simulink model "model_spis"  (R2016b)
settings: Solver=FixedStepDiscrete  StartTime=0.0  StopTime=inf  FixedStep=sampleTime  RelTol=1e-3
PostLoadFcn:
  | parameters_spis;
  | 
  | % set requested state
  | set_param('model_spis/Requested state','Value',num2str(0));
InitFcn:
  | parameters_spis;
  | 
  | % set requested state
  | set_param('model_spis/Requested state','Value',num2str(0));
StartFcn:
  | parameters_spis;
  | 
  | % set requested state
  | set_param('model_spis/Requested state','Value',num2str(0));
undefined symbols (not defined in the file): FM1, FM2, Lb, Lf, Lu, sampleTime
libraries: simulink x29, LibraryFM x14, VariousBlocksLibrary x7, simulink_extras x1
(part 3 of 3)

== matlab function model_spis/Experiment & Haptics/Subsystem3/visuomotor rotation1 ==
  data: xBound input; pos_ref output; yBound input; vel input; pos_ref_prev input; sampleTime parameter; vel_ref output
function [pos_ref, vel_ref] = rotation(xBound, yBound, vel, pos_ref_prev,sampleTime)

persistent velDir;

if isempty(velDir)
    velDir = [1;0]; % initial velocity
end

pos_ref_tmp = pos_ref_prev + velDir*vel*sampleTime;

% check for x boundary
if (pos_ref_tmp(1) > xBound)
    velDir = [0;1];
elseif (pos_ref_tmp(1) < -xBound)
    velDir = [0;-1];
elseif (pos_ref_tmp(2) > yBound)
    velDir = [-1;0];
elseif (pos_ref_tmp(2) < -yBound)
    velDir = [1;0];
end

% forward Euler integration
pos_ref = pos_ref_prev + velDir*vel*sampleTime;
vel_ref = velDir*vel;

end

== matlab function model_spis/Robot1/DataFromEtherCAT/Calculate Arrange Joint and Op Space/forward kinematics1/Je ==
  data: q input; Je output size=[2 2]; Lf parameter; Lu parameter; Lb parameter
function Je = Je( q, Lf, Lu, Lb)
%#codegen

% Calculate the Jacobian for this particular device configuration.
% Note that the function func_eq_Je needs to be in the libraries/kinematis_functions folder

% jacobians
Je = func_eq_Je(q(1),q(2),Lf,Lu,Lb);

== matlab function model_spis/Robot1/DataFromEtherCAT/Calculate Arrange Joint and Op Space/forward kinematics1/Jedot ==
  data: q input; qdot input; Jedot output size=[2 2]; Lf parameter; Lu parameter; Lb parameter
function Jedot = Jedot( q, qdot, Lf, Lu, Lb)
%#codegen

% Calculate the time derivative of the Jacobian for this particular device configuration.
% Note that the function func_eq_Je needs to be in the libraries/kinematis_functions folder


% jacobians
Jedot = func_eq_Jedot(q(1),q(2),qdot(1),qdot(2),Lf,Lu,Lb);

== matlab function model_spis/Robot1/DataFromEtherCAT/Calculate Arrange Joint and Op Space/forward kinematics1/calculate xddot ==
  data: qddot input; qdot input size=[2 1]; J input; xddot output size=[2 1]; Jdot input
function xddot = calc_xddot(qddot, qdot, J, Jdot)
%#codegen

xddot = J*qddot + Jdot*qdot;

== matlab function model_spis/Robot2/Controller_PD/PD + nonlin (op space)/nonlinear compensation ==
  data: J input; Jdot input; qdot input; tau output; RobotStruct parameter
function tau = n(J,Jdot,qdot,RobotStruct)
% mass matrix
phat = RobotStruct.DynModParams;

% select parameters
me = phat(3);
Fs1 = phat(4);
Fv1 = phat(5);
Fs2 = phat(6);
Fv2 = phat(7);

% % jacobians
% J = func_eq_Je(q(1),q(2),Lf,Lu,Lb);
% Jdot = func_eq_Jedot(q(1),q(2),qdot(1),qdot(2),Lf,Lu,Lb);

% calculate joint space mass matrix;
p = [me;Fs1;Fv1;Fs2;Fv2];

% psi 
Psi = [(J'*Jdot)*qdot [ssign(qdot(1)) qdot(1); 0 0] [0 0; ssign(qdot(2)) qdot(2)]];

% torque
tau = Psi*p;

function x = ssign(u,b)
%% x = ssign(u,b)
% soft sign
if nargin < 2
    b = 4;
end

x = 2./(1+exp(-b*u))-1;

== matlab function model_spis/Experiment & Haptics/visuomotor rotation ==
  data: x_home input; x input; y output; theta input; doRotation input
function y = fcn(x_home,x,theta,doRotation)

x = x - x_home;

if (doRotation)
    R = [cos(theta) -sin(theta); 
         sin(theta) cos(theta)];
    y = R*x;
else
    y = x;
end

y = y + x_home;

== matlab function model_spis/Robot1/DataFromEtherCAT/Calculate Arrange Joint and Op Space/forward kinematics/forward kinematics ==
  data: q input; x output size=[2 1]; Lf parameter; Lu parameter; Lb parameter
function x = FK(q, Lf, Lu, Lb)
%#codegen

% Calculate the endpoint position (forward kinematics)
% Note that the function func_eq_FK needs to be in the libraries/kinematis_functions folder


x = func_eq_FK(q(1),q(2),Lf,Lu,Lb);

== matlab function model_spis/Robot1/DataFromEtherCAT/Calculate Arrange Joint and Op Space/forward kinematics1/forward kinematics ==
  data: q input; x output size=[2 1]; Lf parameter; Lu parameter; Lb parameter
function x = FK(q, Lf, Lu, Lb)
%#codegen

% Calculate the endpoint position (forward kinematics)
% Note that the function func_eq_FK needs to be in the libraries/kinematis_functions folder


x = func_eq_FK(q(1),q(2),Lf,Lu,Lb);

== matlab function model_spis/Robot1/DataToEtherCAT/FTSensorError/MATLAB Function ==
  data: ForcesTorques input; e output; MaxForcesTorques input
function e = fcn(ForcesTorques, MaxForcesTorques)

% throw error when any of the forces/torques go over a max allowable value
if any(abs(ForcesTorques) > MaxForcesTorques) 
    e = 1;
else
    e = 0;
end

== matlab function model_spis/Robot1/Controller_PD/PD + nonlin (op space)/invJ1 ==
  data: x input; J input; y output
function y = invJ(x,J)

y = J.'*x;

== matlab function model_spis/Robot2/DataFromEtherCAT/Calculate Arrange Joint and Op Space/Condition number ==
  data: J input; C output
function C = conditioning(J)
%#codegen

C = norm(J)*norm(pinv(J));

== matlab function model_spis/Robot2/DataFromEtherCAT/Calculate Arrange Joint and Op Space/IK all joints ==
  data: x input; q_all output; Lf parameter; Lu parameter; Lb parameter
function q_all = IK_all(x,Lf,Lu,Lb)
%#codegen

q_all = func_eqs_IK_all(x(1),x(2),Lf,Lu,Lb);

if any(isnan(q_all)) || any(isinf(q_all))
    q_all = zeros(5,1);
end

== matlab function model_spis/Robot2/DataFromEtherCAT/Calculate Arrange Joint and Op Space/forward kinematics/Je ==
  data: q input; Je output size=[2 2]; Lf parameter; Lu parameter; Lb parameter
function Je = Je( q, Lf, Lu, Lb)
%#codegen

% Calculate the Jacobian for this particular device configuration.
% Note that the function func_eq_Je needs to be in the libraries/kinematis_functions folder

% jacobians
Je = func_eq_Je(q(1),q(2),Lf,Lu,Lb);

== matlab function model_spis/Experiment & Haptics/visuomotor rotation1 ==
  data: x_home input; x input; y output; theta input; doRotation input
function y = fcn(x_home,x,theta,doRotation)

x = x - x_home;

if (doRotation)
    R = [cos(theta) -sin(theta); 
         sin(theta) cos(theta)];
    y = R*x;
else
    y = x;
end

y = y + x_home;

== matlab function model_spis/Robot2/DataFromEtherCAT/Calculate Arrange Joint and Op Space/forward kinematics/Jedot ==
  data: q input; qdot input; Jedot output size=[2 2]; Lf parameter; Lu parameter; Lb parameter
function Jedot = Jedot( q, qdot, Lf, Lu, Lb)
%#codegen

% Calculate the time derivative of the Jacobian for this particular device configuration.
% Note that the function func_eq_Je needs to be in the libraries/kinematis_functions folder


% jacobians
Jedot = func_eq_Jedot(q(1),q(2),qdot(1),qdot(2),Lf,Lu,Lb);

== matlab function model_spis/Robot1/DataFromEtherCAT/Calculate Arrange Joint and Op Space/forward kinematics/Je ==
  data: q input; Je output size=[2 2]; Lf parameter; Lu parameter; Lb parameter
function Je = Je( q, Lf, Lu, Lb)
%#codegen

% Calculate the Jacobian for this particular device configuration.
% Note that the function func_eq_Je needs to be in the libraries/kinematis_functions folder

% jacobians
Je = func_eq_Je(q(1),q(2),Lf,Lu,Lb);

== matlab function model_spis/Robot1/DataFromEtherCAT/Calculate Arrange Joint and Op Space/forward kinematics/Jedot ==
  data: q input; qdot input; Jedot output size=[2 2]; Lf parameter; Lu parameter; Lb parameter
function Jedot = Jedot( q, qdot, Lf, Lu, Lb)
%#codegen

% Calculate the time derivative of the Jacobian for this particular device configuration.
% Note that the function func_eq_Je needs to be in the libraries/kinematis_functions folder


% jacobians
Jedot = func_eq_Jedot(q(1),q(2),qdot(1),qdot(2),Lf,Lu,Lb);

== matlab function model_spis/Robot1/DataFromEtherCAT/FTSensor_K6D27/CorrectOffset ==
  data: u_in input; u_out output; reset input; corrected output
function [u_out,corrected] = CorrectOffset(u_in,reset)
%#codegen

persistent data_ offset_ counter_ corrected_;
N = 1000;

% initialize
if isempty(data_)
    data_ = zeros(size(u_in,1), N);
    offset_ = zeros(size(u_in));
    counter_ = 1;
    corrected_ = 0;
end

if (counter_ <= N)
    data_(:,counter_) = u_in;
end

counter_ = counter_ + 1;
if reset
    counter_ = 1;
end

% calculate mean
if counter_ == N
    corrected_ = 1;
    offset_ = mean(data_,2);
end

corrected = corrected_;
u_out = u_in - offset_;

== matlab function model_spis/Robot2/DataFromEtherCAT/Calculate Arrange Joint and Op Space/forward kinematics/calculate xddot ==
  data: qddot input; qdot input size=[2 1]; J input; xddot output size=[2 1]; Jdot input
function xddot = calc_xddot(qddot, qdot, J, Jdot)
%#codegen

xddot = J*qddot + Jdot*qdot;

== matlab function model_spis/Robot1/DataFromEtherCAT/Calculate Arrange Joint and Op Space/IK all joints ==
  data: x input; q_all output; Lf parameter; Lu parameter; Lb parameter
function q_all = IK_all(x,Lf,Lu,Lb)
%#codegen

q_all = func_eqs_IK_all(x(1),x(2),Lf,Lu,Lb);

if any(isnan(q_all)) || any(isinf(q_all))
    q_all = zeros(5,1);
end

== matlab function model_spis/Robot1/DataFromEtherCAT/Calculate Arrange Joint and Op Space/forward kinematics/calculate xddot ==
  data: qddot input; qdot input size=[2 1]; J input; xddot output size=[2 1]; Jdot input
function xddot = calc_xddot(qddot, qdot, J, Jdot)
%#codegen

xddot = J*qddot + Jdot*qdot;

== matlab function model_spis/Robot2/DataFromEtherCAT/Calculate Arrange Joint and Op Space/forward kinematics/forward kinematics ==
  data: q input; x output size=[2 1]; Lf parameter; Lu parameter; Lb parameter
function x = FK(q, Lf, Lu, Lb)
%#codegen

% Calculate the endpoint position (forward kinematics)
% Note that the function func_eq_FK needs to be in the libraries/kinematis_functions folder


x = func_eq_FK(q(1),q(2),Lf,Lu,Lb);

== matlab function model_spis/Robot1/Controller_PD/PD + nonlin (op space)/nonlinear compensation ==
  data: J input; Jdot input; qdot input; tau output; RobotStruct parameter
function tau = n(J,Jdot,qdot,RobotStruct)
% mass matrix
phat = RobotStruct.DynModParams;

% select parameters
me = phat(3);
Fs1 = phat(4);
Fv1 = phat(5);
Fs2 = phat(6);
Fv2 = phat(7);

% % jacobians
% J = func_eq_Je(q(1),q(2),Lf,Lu,Lb);
% Jdot = func_eq_Jedot(q(1),q(2),qdot(1),qdot(2),Lf,Lu,Lb);

% calculate joint space mass matrix;
p = [me;Fs1;Fv1;Fs2;Fv2];

% psi 
Psi = [(J'*Jdot)*qdot [ssign(qdot(1)) qdot(1); 0 0] [0 0; ssign(qdot(2)) qdot(2)]];

% torque
tau = Psi*p;

function x = ssign(u,b)
%% x = ssign(u,b)
% soft sign
if nargin < 2
    b = 8;
end

x = 2./(1+exp(-b*u))-1;

== matlab function model_spis/Robot2/DataFromEtherCAT/Calculate Arrange Joint and Op Space/forward kinematics1/Je ==
  data: q input; Je output size=[2 2]; Lf parameter; Lu parameter; Lb parameter
function Je = Je( q, Lf, Lu, Lb)
%#codegen

% Calculate the Jacobian for this particular device configuration.
% Note that the function func_eq_Je needs to be in the libraries/kinematis_functions folder

% jacobians
Je = func_eq_Je(q(1),q(2),Lf,Lu,Lb);

== matlab function model_spis/Robot2/DataFromEtherCAT/Calculate Arrange Joint and Op Space/forward kinematics1/Jedot ==
  data: q input; qdot input; Jedot output size=[2 2]; Lf parameter; Lu parameter; Lb parameter
function Jedot = Jedot( q, qdot, Lf, Lu, Lb)
%#codegen

% Calculate the time derivative of the Jacobian for this particular device configuration.
% Note that the function func_eq_Je needs to be in the libraries/kinematis_functions folder


% jacobians
Jedot = func_eq_Jedot(q(1),q(2),qdot(1),qdot(2),Lf,Lu,Lb);

== matlab function model_spis/Robot2/DataFromEtherCAT/Calculate Arrange Joint and Op Space/forward kinematics1/calculate xddot ==
  data: qddot input; qdot input size=[2 1]; J input; xddot output size=[2 1]; Jdot input
function xddot = calc_xddot(qddot, qdot, J, Jdot)
%#codegen

xddot = J*qddot + Jdot*qdot;

== matlab function model_spis/Robot2/DataFromEtherCAT/Calculate Arrange Joint and Op Space/forward kinematics1/forward kinematics ==
  data: q input; x output size=[2 1]; Lf parameter; Lu parameter; Lb parameter
function x = FK(q, Lf, Lu, Lb)
%#codegen

% Calculate the endpoint position (forward kinematics)
% Note that the function func_eq_FK needs to be in the libraries/kinematis_functions folder


x = func_eq_FK(q(1),q(2),Lf,Lu,Lb);

== matlab function model_spis/Robot2/DataFromEtherCAT/FTSensor_K6D27/CorrectOffset ==
  data: u_in input; u_out output; reset input; corrected output
function [u_out,corrected] = CorrectOffset(u_in,reset)
%#codegen

persistent data_ offset_ counter_ corrected_;
N = 1000;

% initialize
if isempty(data_)
    data_ = zeros(size(u_in,1), N);
    offset_ = zeros(size(u_in));
    counter_ = 1;
    corrected_ = 0;
end

if (counter_ <= N)
    data_(:,counter_) = u_in;
end

counter_ = counter_ + 1;
if reset
    counter_ = 1;
end

% calculate mean
if counter_ == N
    corrected_ = 1;
    offset_ = mean(data_,2);
end

corrected = corrected_;
u_out = u_in - offset_;

== matlab function model_spis/Experiment & Haptics/isAtTarget ==
  data: cursorPos input; atTarget output; targetPos input
function atTarget = isAtTarget(cursorPos, targetPos)

if (norm(cursorPos-targetPos) < 0.003)
    atTarget = 1;
else
    atTarget = 0;
end

== matlab function model_spis/Robot2/DataFromEtherCAT/FTSensor_K6D27/SensorToOperationalSpace ==
  data: q_all input; Fs input; FTOpSpace output; transmatside input
function FTOpSpace = ForceSensorToOperationalSpace(q_all,Fs,transmatside)
%#codegen
q1 = q_all(1);
q2 = q_all(2);
q4 = q_all(4);
q5 = q_all(5);

% based on which arm the force sensor is connected
switch transmatside
    case 1
        alpha = pi-q2;   
        beta = q1+alpha-pi/2;
        R0 = rotmat(beta);
        R = blkdiag(R0,R0); % transform forces and moments
    case 2
        alpha = -(pi - q4);
        beta = q5+alpha-pi/2;
        R0 = rotmat(beta);
        R = blkdiag(R0,R0); % transform forces and moments
    otherwise
        R = eye(length(Fs));
end

% transform force
FTOpSpace = R*Fs;

function R = rotmat(q)

R = [cos(q) -sin(q) 0;...
      sin(q)  cos(q) 0;...
      0       0      1];

== matlab function model_spis/Robot2/DataToEtherCAT/CreateSingleErrorValue1/ErrorToPower2 ==
  data: u input; e output
function e = errorToPowerOf2(u)

e = (2.^(0:length(u)-1))*u;

== matlab function model_spis/Robot2/DataToEtherCAT/CreateSingleErrorValue2/ErrorToPower2 ==
  data: u input; e output
function e = errorToPowerOf2(u)

e = (2.^(0:length(u)-1))*u;

== matlab function model_spis/Robot2/DataToEtherCAT/FTSensorError/MATLAB Function ==
  data: ForcesTorques input; e output; MaxForcesTorques input
function e = fcn(ForcesTorques, MaxForcesTorques)

% throw error when any of the forces/torques go over a max allowable value
if any(abs(ForcesTorques) > MaxForcesTorques) 
    e = 1;
else
    e = 0;
end

== matlab function model_spis/Robot2/DataToEtherCAT/WorkspacePositionGuard/CheckInternalAngles ==
  data: theta input; angleError output
function angleError = checkInternalErrors(theta)
%#codegen


angleError = 0;
if any(theta([2 4]) >= 0.95*pi)
    angleError = 1;
end

== matlab function model_spis/Robot2/DataToEtherCAT/WorkspacePositionGuard/EndpointPositionGuard ==
  data: correctState input; xe input; error output
function error = fcn(correctState, xe)
%#codegen


error = 0;

% only check workspace boundaries after homing state is done
if ~correctState 
    return; 
end

% x0 = 0;
% y0 = 0.2354;
% a = 0.11;
% b = 0.08;

% workspace (see design document)
x0 = 0;
y0 = 0.25024;
a = 0.1746;
b = 0.13;%0.1048;

% check if endpoint is outside a predefined ellipse
x = xe(1);
y = xe(2);

% workspace is defined as an ellipse
e = (x-x0)^2 / a^2 + (y-y0)^2 / b^2;

% if is larger than 1, the endpoint is outside the workspace
if e > 1
    error = 1;
end

== matlab function model_spis/Experiment & Haptics/Admittance // Virtual model/Admittance_BROS1/Virtual model ==
  data: lim_pos output; lim_vel output; lim_acc output; x1 output size=[2 1]; xdot1 output; xddot1 output; M_v input; B_v input; F input; x0 input; x_nompos input; x1_prev input size=2; xdot1_prev input size=2
function [lim_pos,lim_vel,lim_acc,x1,xdot1,xddot1] = AC(M_v, B_v, F, x0, x_nompos, x1_prev, xdot1_prev)


Ts = 0.001;
maxRadius = 0.1;
maxVel = 2.0;
maxAcc = 100.0;

persistent x1_prev_tmp;
if isempty(x1_prev_tmp)
    x1_prev_tmp = x0;
else
    x1_prev_tmp = x1_prev;
end

% lower bounds to 
m_v = max(0.01,M_v); %lower bound M_v = 1 kg
b_v = max(0,B_v);

% semi-implicit Euler integration
xddot1 = (F - b_v*xdot1_prev)/m_v;
[xddot1, lim_acc] = limit(xddot1,maxAcc);

xdot1 = xdot1_prev + xddot1*Ts;
[xdot1,lim_vel] = limit(xdot1,maxVel);

if (lim_vel)
    xddot1 = [0;0];
end

x1 = x1_prev_tmp + xdot1*Ts;

[x1,lim_pos] = limit(x1-x_nompos,maxRadius);
if (lim_pos)
    unitVec = x1/norm(x1);
    xdot1 = xdot1 - dot(unitVec,xdot1)*unitVec;     % remove normal component
    xddot1 = xddot1 - dot(unitVec,xddot1)*unitVec;  % remove normal component 
end
x1 = x1 + x_nompos;

end

function [y,lim] = limit(x,maxVal)
    vecLen = norm(x);
    if vecLen > maxVal
        y = x / vecLen * maxVal;
        lim = 1; 
    else
        y = x;
        lim = 0;
    end
end

== matlab function model_spis/Experiment & Haptics/Admittance/Virtual model ==
  data: x1 output size=[2 1]; xdot1 output; xddot1 output; M_v input; B_v input; F1 input; x1_0 input; F2 input; x2_0 input; x_nompos input; x1_prev input size=2; xdot1_prev input size=2; x2_prev input; xdot2_prev input; x2 output; xdot2 output; xddot2 output
function [x1,xdot1,xddot1,x2,xdot2,xddot2] = AC(M_v,B_v,F1,x1_0,F2, x2_0,x_nompos,x1_prev,xdot1_prev,x2_prev,xdot2_prev)
%% function [x1,xdot1,xddot1,x2,xdot2,xddot2] = AC(M_v,B_v,F1,x1_0,F2, x2_0,x_nompos,x1_prev,xdot1_prev,x2_prev,xdot2_prev)
%
%

persistent x1_prev_tmp;
persistent x2_prev_tmp;
if isempty(x1_prev_tmp)
    x1_prev_tmp = x1_0;
else
    x1_prev_tmp = x1_prev; 
end
if isempty(x2_prev_tmp) 
    x2_prev_tmp = x2_0;
else
    x2_prev_tmp = x2_prev; 
end

% parameters
Ts = 0.001;
maxRadius = 0.1;
maxVel = 2.0;
maxAcc = 100.0;

% lower bounds to 
m_v = max(0.2,M_v); %lower bound M_v = 1 kg
b_v = max(0,B_v);

% semi-implicit Euler integration

% acceleration
xddot1 = (F1 - b_v*xdot1_prev)/m_v;
[xddot1, ~] = limit(xddot1,maxAcc);

xddot2 = (F2 - b_v*xdot2_prev)/m_v;
[xddot2, ~] = limit(xddot2,maxAcc);

% velocity
xdot1 = xdot1_prev + xddot1*Ts;
[xdot1,lim_vel] = limit(xdot1,maxVel);
if (lim_vel), xddot1 = [0;0]; end

xdot2 = xdot2_prev + xddot2*Ts;
[xdot2,lim_vel] = limit(xdot2,maxVel);
if (lim_vel), xddot2 = [0;0]; end

% position
x1 = x1_prev_tmp + xdot1*Ts;
[x1,lim_pos] = limit(x1-x_nompos,maxRadius);
if (lim_pos)
    unitVec = x1/norm(x1);
    xdot1 = xdot1 - dot(unitVec,xdot1)*unitVec;     % remove normal component
    xddot1 = xddot1 - dot(unitVec,xddot1)*unitVec;  % remove normal component
end
x1 = x1 + x_nompos;

x2 = x2_prev_tmp + xdot2*Ts;
[x2,lim_pos] = limit(x2-x_nompos,maxRadius);
if (lim_pos)
    unitVec = x2/norm(x2);
    xdot2 = xdot2 - dot(unitVec,xdot2)*unitVec;     % remove normal component
    xddot2 = xddot2 - dot(unitVec,xddot2)*unitVec;  % remove normal component
end
x2 = x2 + x_nompos;

end

function [y,lim] = limit(x,maxVal)
%% function [y,lim] = limit(x,maxVal)
% limit vector

vecLen = norm(x);
if vecLen > maxVal
    y = x / vecLen * maxVal;
    lim = 1; 
else
    y = x;
    lim = 0;
end

end

== matlab function model_spis/Robot1/DataToEtherCAT/CreateSingleErrorValue2/ErrorToPower2 ==
  data: u input; e output
function e = errorToPowerOf2(u)

e = (2.^(0:length(u)-1))*u;

== matlab function model_spis/Robot1/DataToEtherCAT/CreateSingleErrorValue1/ErrorToPower2 ==
  data: u input; e output
function e = errorToPowerOf2(u)

e = (2.^(0:length(u)-1))*u;

== matlab function model_spis/Experiment & Haptics/Admittance // Virtual model/Virtual Spring ==
  data: isConnected input; Fs1_2 output; Fs2_1 output; Kp input; Kd input; x1 input; xdot1 input; x2 input; xdot2 input size=2
function [Fs1_2, Fs2_1] = Fs(isConnected, Kp, Kd, x1, xdot1, x2, xdot2)
maxForce = 20;

% spring force 1
if isConnected
    Fs1_2 = Kp*(x2-x1) + Kd*(xdot2-xdot1);
    Fs1_2 = limit(Fs1_2,maxForce);
else
    Fs1_2 = [0;0];
end

% spring force 2
if isConnected
    Fs2_1 = Kp*(x1-x2) + Kd*(xdot1-xdot2);
    Fs2_1 = limit(Fs2_1,maxForce);
else
    Fs2_1 = [0;0];
end

end

function [y,lim] = limit(x,maxVal)
    vecLen = norm(x);
    if vecLen > maxVal
        y = x / vecLen * maxVal;
        lim = 1; 
    else
        y = x;
        lim = 0;
    end
end

== matlab function model_spis/Robot1/DataFromEtherCAT/FTSensor_K6D27/SensorToOperationalSpace ==
  data: q_all input; Fs input; FTOpSpace output; transmatside input
function FTOpSpace = ForceSensorToOperationalSpace(q_all,Fs,transmatside)
%#codegen
q1 = q_all(1);
q2 = q_all(2);
q4 = q_all(4);
q5 = q_all(5);

% based on which arm the force sensor is connected
switch transmatside
    case 1
        alpha = pi-q2;   
        beta = q1+alpha-pi/2;
        R0 = rotmat(beta);
        R = blkdiag(R0,R0); % transform forces and moments
    case 2
        alpha = -(pi - q4);
        beta = q5+alpha-pi/2;
        R0 = rotmat(beta);
        R = blkdiag(R0,R0); % transform forces and moments
    otherwise
        R = eye(length(Fs));
end

% transform force
FTOpSpace = R*Fs;

function R = rotmat(q)

R = [cos(q) -sin(q) 0;...
      sin(q)  cos(q) 0;...
      0       0      1];

== matlab function model_spis/Experiment & Haptics/Admittance // Virtual model/Admittance_BROS1/Virtual model1 ==
  data: B_v_spis output size=1; M_v input; B_v_max input; F_meas input; v_d input; x_dot_meas input; E_hr_prev input; E_hr output size=1; a input
function [B_v_spis ,E_hr] = AC(M_v, B_v_max, F_meas, v_d, x_dot_meas, E_hr_prev, a)
    T_s = 0.001;
    E_hr = E_hr_prev + dot(x_dot_meas,F_meas)*T_s;
    H = 0.5*M_v*dot(v_d,v_d);
    B_v_spis = (0.5+0.5*tanh(a*(H - E_hr))) * B_v_max; % double(H >= E_hr)   B_v_max
end

== matlab function model_spis/Robot1/DataToEtherCAT/WorkspacePositionGuard/CheckInternalAngles ==
  data: theta input; angleError output
function angleError = checkInternalErrors(theta)
%#codegen


angleError = 0;
if any(theta([2 4]) >= 0.95*pi)
    angleError = 1;
end

== matlab function model_spis/Robot1/DataToEtherCAT/WorkspacePositionGuard/EndpointPositionGuard ==
  data: correctState input; xe input; error output
function error = fcn(correctState, xe)
%#codegen


error = 0;

% only check workspace boundaries after homing state is done
if ~correctState 
    return; 
end

% x0 = 0;
% y0 = 0.2354;
% a = 0.11;
% b = 0.08;

% workspace (see design document)
x0 = 0;
y0 = 0.25024;
a = 0.1746;
b = 0.13;%0.1048;

% check if endpoint is outside a predefined ellipse
x = xe(1);
y = xe(2);

% workspace is defined as an ellipse
e = (x-x0)^2 / a^2 + (y-y0)^2 / b^2;

% if is larger than 1, the endpoint is outside the workspace
if e > 1
    error = 1;
end
